simulink model "ModelSupervisor"  (R2017b)
settings: Solver=ode3  StartTime=0.0  StopTime=T_max  FixedStep=h  RelTol=1e-3
values from neighbouring files (symbols this model uses):
  b = 0.1    [Input_LQR.m]    (also in TestKalman.m; TestSuper.m; TestVahidComparison.m; parameter.m)
  C_sup = [1 0 0 0 0 0 ... (first row only)    [TestSuper.m]
  delta = cell(1,length(L_sup))    [TestSuper.m]
  g = 9.81    [Input_LQR.m]    (also in TestKalman.m; TestSuper.m; TestVahidComparison.m; parameter.m = 9.8)
  gamma = cell(1,length(L_sup))    [TestSuper.m]
  h = 0.01    [Input_LQR.m]    (also in TestKalman.m; TestSuper.m = 0.001; TestVahidComparison.m = 0.001; parameter.m)
  K = lqr(A, B, Q, R)    [Input_LQR.m]    (also in TestKalman.m; TestSuper.m)
  k = 0.15    [Input_LQR.m]    (also in TestKalman.m; TestSuper.m; TestVahidComparison.m; parameter.m)
  L = 1.4    [Input_LQR.m]    (also in TestKalman.m; TestSuper.m = 1.025; TestVahidComparison.m)
  L_2 = 1.525    [TestSuper.m]
  M = 1    [Input_LQR.m]    (also in TestKalman.m; TestSuper.m; TestVahidComparison.m; parameter.m)
  m = 3/4    (= 0.75)    [Input_LQR.m]    (also in TestKalman.m; TestSuper.m; TestVahidComparison.m; parameter.m)
  P_0 = diag([1,1,1,1,100,100])    [Input_LQR.m]    (also in TestKalman.m = diag([1,1,1,1,100,100])*0.001; TestSuper.m = diag([1,1,1,1,100,100])*0.001)
  phi = cell(1,length(L_sup))    [TestSuper.m]
  Q_kalman = diag([10, 10e-4])    [Input_LQR.m]    (also in TestKalman.m = diag([(10), (10e-4)]); TestSuper.m = diag([(10), (10e-4)]))
  R_kalman = diag([(10e-7), (10e-7)])    [Input_LQR.m]    (also in TestKalman.m; TestSuper.m)
  R_sup = R_kalman    [TestSuper.m]
  sys1 = c2d(ss(A_kA1, B_kA1, C_kA1, D_kA1), h)    [TestSuper.m]
  sys2 = c2d(ss(A_kA2, B_kA2, C_kA2, D_kA2), h)    [TestSuper.m]
  sys3 = c2d(ss(A_kA3, B_kA3, C_kA3, D_kA3), h)    [TestSuper.m]
  sys4 = c2d(ss(A_kA4, B_kA4, C_kA4, D_kA4), h)    [TestSuper.m]
  theta_0 = 0    [Input_LQR.m]    (also in TestKalman.m = 0.1; TestSuper.m = 0.1; TestVahidComparison.m = 0.1)
  theta_dot0 = 0    [Input_LQR.m]    (also in TestKalman.m; TestSuper.m; TestVahidComparison.m)
  X_0 = [0 0 0 0 0 0]'    [Input_LQR.m]    (also in TestKalman.m = [x_0 theta_0 x_dot0 theta_dot0 0 0]'; TestSuper.m = [x_0 theta_0 x_dot0 theta_dot0 0 0]')
  x_0 = 0    [Input_LQR.m]    (also in TestKalman.m; TestSuper.m; TestVahidComparison.m)
  x_dot0 = 0    [Input_LQR.m]    (also in TestKalman.m; TestSuper.m; TestVahidComparison.m)
  y_0 = [0 0]    [Input_LQR.m]    (also in TestKalman.m; TestSuper.m)
undefined symbols (not defined in the file or in its folder): A_kA1, A_kA2, A_kA3, A_kA4, B_kA1, B_kA2, B_kA3, B_kA4, C_kA1, C_kA2, C_kA3, C_kA4, D_kA1, D_kA2, D_kA3, D_kA4
libraries: simulink x6
settings Model: Creator=Erik  LastModifiedBy=Andreas
settings DataIOCC: LimitDataPoints=on  SaveFormat=Array
settings OptimizationCC: BlockReduction=off  BooleanDataType=off  LifeSpan=inf
settings DebuggingCC: SaveWithParameterizedLinksMsg=none  UnderspecifiedInitializationDetection=Classic  MergeDetectMultiDrivingBlocksExec=none  SignalResolutionControl=TryResolveAllWithWarning  SFUnexpectedBacktrackingDiag=warning  SFNoUnconditionalDefaultTransitionDiag=warning  SFExecutionAtInitializationDiag=none
settings HardwareCC: ProdBitPerPointer=32  ProdBitPerSizeT=32  ProdBitPerPtrDiffT=32  ProdLargestAtomicFloat=None  ProdIntDivRoundTo=Undefined  ProdEndianess=Unspecified  ProdWordSize=32  ProdHWDeviceType=32-bit Generic  TargetUnknown=on
settings ModelReferenceCC: PropagateSignalLabelsOutOfModel=off
settings CodeAppCC: StateflowObjectComments=on
settings GRTTargetCC: TargetLangStandard=C89/C90 (ANSI)  GeneratePreprocessorConditionals=Disable all
settings ConfigComp: CovMetricSettings=dw  CovHtmlReporting=on  CovSaveCumulativeToWorkspaceVar=on  CovSaveSingleToWorkspaceVar=on  CovExternalEMLEnable=off  CovSFcnEnable=off

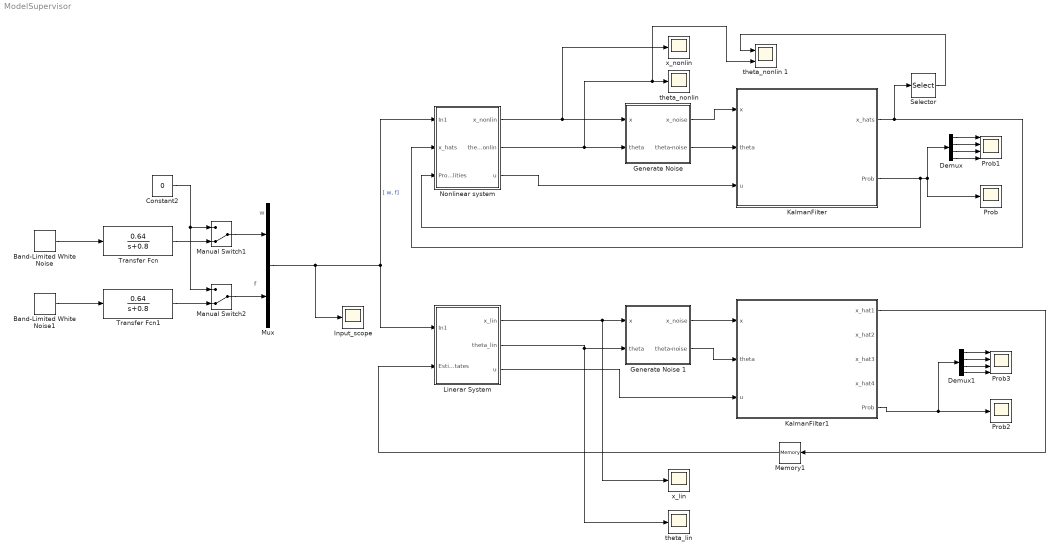
== system ModelSupervisor ==
  note: f
  note: w
  Band-Limited White Noise : simulink/Sources/Band-Limited White Noise  Cov=Q_kalman(1,1)  Ts=h  seed=[23343]
  Band-Limited White Noise1 : simulink/Sources/Band-Limited White Noise  Cov=Q_kalman(2,2)  Ts=h  seed=[23344]
  Constant2 : Constant  Value=0
  Demux : Demux
  Demux1 : Demux
  "Generate Noise " : Subsystem
  Generate Noise 1 : Subsystem
  Input_scope : Scope
  KalmanFilter : Subsystem
  KalmanFilter1 : Subsystem
  Linerar System : Subsystem
  Manual Switch1 : ManualSwitch  CurrentSetting=0
  Manual Switch2 : ManualSwitch  CurrentSetting=0
  Memory1 : Memory  InitialCondition=X_0
  Mux : Mux  Inputs=2
  "Nonlinear system " : Subsystem
  Prob : Scope
  Prob1 : Scope  NumInputPorts=4
  Prob2 : Scope
  Prob3 : Scope  NumInputPorts=4
  Selector : Selector  InputPortWidth=24  IndexOptions=Index vector (dialog)  Indices=[2 7 13 19]  OutputSizes=1
  Transfer Fcn : TransferFcn  Numerator=[0.64]  Denominator=[1 0.8]
  Transfer Fcn1 : TransferFcn  Numerator=[0.64]  Denominator=[1 0.8]
  theta_lin : Scope
  "theta_nonlin " : Scope
  theta_nonlin 1 : Scope  NumInputPorts=2
  x_lin : Scope
  x_nonlin : Scope
  wires:
  Mux/1 -> Linerar System/1(In1), "Nonlinear system "/1(In1), Input_scope/1  "[ w, f]"
  "Nonlinear system "/1(x_nonlin) -> x_nonlin/1, "Generate Noise "/1(x)
  "Nonlinear system "/2(theta_nonlin) -> theta_nonlin 1/2, "theta_nonlin "/1, "Generate Noise "/2(theta)
  Linerar System/2(theta_lin) -> theta_lin/1, Generate Noise 1/2(theta)
  "Nonlinear system "/3(u) -> KalmanFilter/3("u ")
  KalmanFilter/1(x_hats) -> Selector/1, "Nonlinear system "/2(x_hats)
  Band-Limited White Noise/1 -> Transfer Fcn/1
  Band-Limited White Noise1/1 -> Transfer Fcn1/1
  Transfer Fcn/1 -> Manual Switch1/2
  "Generate Noise "/1(x_noise) -> KalmanFilter/1(x)
  "Generate Noise "/2(theta-noise) -> KalmanFilter/2(theta)
  Generate Noise 1/2(theta-noise) -> KalmanFilter1/2(theta)
  Linerar System/3(u) -> KalmanFilter1/3("u ")
  Linerar System/1(x_lin) -> x_lin/1, Generate Noise 1/1(x)
  Generate Noise 1/1(x_noise) -> KalmanFilter1/1(x)
  Memory1/1 -> Linerar System/2(Estimated states)
  KalmanFilter/2(Prob) -> "Nonlinear system "/3(Probabilities), Prob/1, Demux/1
  KalmanFilter1/1(x_hat1) -> Memory1/1
  Demux/1 -> Prob1/1
  Demux/2 -> Prob1/2
  Demux/3 -> Prob1/3
  Demux/4 -> Prob1/4
  KalmanFilter1/5(Prob) -> Demux1/1, Prob2/1
  Demux1/1 -> Prob3/1
  Demux1/2 -> Prob3/2
  Demux1/3 -> Prob3/3
  Demux1/4 -> Prob3/4
  Manual Switch1/1 -> Mux/1
  Constant2/1 -> Manual Switch2/1, Manual Switch1/1
  Transfer Fcn1/1 -> Manual Switch2/2
  Manual Switch2/1 -> Mux/2
  Selector/1 -> theta_nonlin 1/1

== system ModelSupervisor/Generate Noise  ==
  x : Inport
  theta : Inport  Port=2
  Band-Limited White Noise2 : simulink/Sources/Band-Limited White Noise  Cov=R_kalman(1,1)  Ts=h  seed=[23342]
  Band-Limited White Noise3 : simulink/Sources/Band-Limited White Noise  Cov=R_kalman(2,2)  Ts=h  seed=[23341]
  Constant : Constant  Value=0
  Manual Switch : ManualSwitch  CurrentSetting=0
  Manual Switch1 : ManualSwitch  CurrentSetting=0
  Sum : Sum  Inputs=++|
  Sum1 : Sum  Inputs=|++
  x_noise : Outport
  theta-noise : Outport  Port=2
  wires:
  Sum/1 -> x_noise/1
  x/1 -> Sum/2
  Band-Limited White Noise2/1 -> Manual Switch1/1
  theta/1 -> Sum1/1
  Sum1/1 -> theta-noise/1
  Band-Limited White Noise3/1 -> Manual Switch/1
  Manual Switch/1 -> Sum1/2
  Manual Switch1/1 -> Sum/1
  Constant/1 -> Manual Switch/2, Manual Switch1/2

== system ModelSupervisor/Generate Noise 1 ==
  x : Inport
  theta : Inport  Port=2
  Band-Limited White Noise2 : simulink/Sources/Band-Limited White Noise  Cov=R_kalman(1,1)  Ts=h  seed=[23342]
  Band-Limited White Noise3 : simulink/Sources/Band-Limited White Noise  Cov=R_kalman(2,2)  Ts=h  seed=[23341]
  Sum : Sum  Inputs=++|
  Sum1 : Sum  Inputs=|++
  x_noise : Outport
  theta-noise : Outport  Port=2
  wires:
  Sum/1 -> x_noise/1
  x/1 -> Sum/2
  Band-Limited White Noise2/1 -> Sum/1
  theta/1 -> Sum1/1
  Sum1/1 -> theta-noise/1
  Band-Limited White Noise3/1 -> Sum1/2

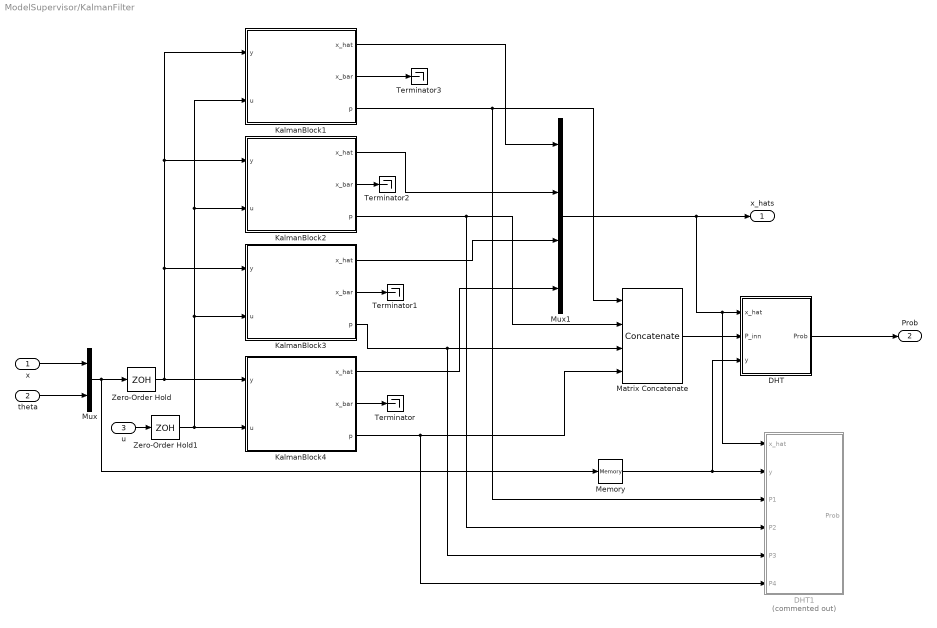
== system ModelSupervisor/KalmanFilter ==
  x : Inport
  theta : Inport  Port=2
  "u " : Inport  Port=3
  DHT : Subsystem
  DHT1 : Subsystem  Commented=on
  KalmanBlock1 : Subsystem
  KalmanBlock2 : Subsystem
  KalmanBlock3 : Subsystem
  KalmanBlock4 : Subsystem
  Matrix Concatenate : Concatenate  NumInputs=4  Mode=Multidimensional array  ConcatenateDimension=2
  Memory : Memory  InitialCondition=[x_0 theta_0]
  Mux : Mux  Inputs=2
  Mux1 : Mux
  Terminator{,1..3} (4 alike) : Terminator
  Zero-Order Hold : ZeroOrderHold  SampleTime=h
  Zero-Order Hold1 : ZeroOrderHold  SampleTime=h
  x_hats : Outport
  Prob : Outport  Port=2
  wires:
  Mux/1 -> Zero-Order Hold/1, Memory/1
  "u "/1 -> Zero-Order Hold1/1
  x/1 -> Mux/1
  theta/1 -> Mux/2
  KalmanBlock4/2(x_bar) -> Terminator/1
  KalmanBlock3/2(x_bar) -> Terminator1/1
  KalmanBlock2/2(x_bar) -> Terminator2/1
  KalmanBlock1/2(x_bar) -> Terminator3/1
  KalmanBlock1/1(x_hat) -> Mux1/1
  KalmanBlock2/1(x_hat) -> Mux1/2
  KalmanBlock3/1(x_hat) -> Mux1/3
  KalmanBlock4/1(x_hat) -> Mux1/4
  DHT/1(Prob) -> Prob/1
  Mux1/1 -> x_hats/1, DHT1/1(x_hat), DHT/1(x_hat)
  KalmanBlock3/3(p) -> DHT1/5(P3), Matrix Concatenate/3
  KalmanBlock2/3(p) -> DHT1/4(P2), Matrix Concatenate/2
  KalmanBlock1/3(p) -> DHT1/3(P1), Matrix Concatenate/1
  Matrix Concatenate/1 -> DHT/2(P_inn)
  Memory/1 -> DHT1/2(y), DHT/3(y)
  KalmanBlock4/3(p) -> DHT1/6(P4), Matrix Concatenate/4
  Zero-Order Hold/1 -> KalmanBlock1/1("y "), KalmanBlock2/1("y "), KalmanBlock3/1("y "), KalmanBlock4/1("y ")
  Zero-Order Hold1/1 -> KalmanBlock1/2("u "), KalmanBlock2/2("u "), KalmanBlock3/2("u "), KalmanBlock4/2("u ")

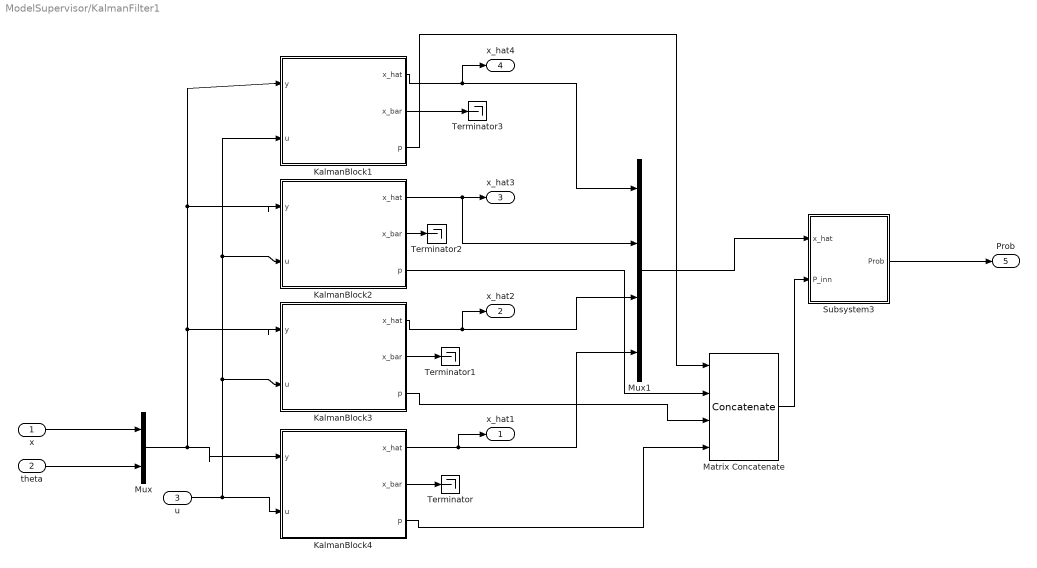
== system ModelSupervisor/KalmanFilter1 ==
  x : Inport
  theta : Inport  Port=2
  "u " : Inport  Port=3
  KalmanBlock1 : Subsystem
  KalmanBlock2 : Subsystem
  KalmanBlock3 : Subsystem
  KalmanBlock4 : Subsystem
  Matrix Concatenate : Concatenate  NumInputs=4  Mode=Multidimensional array  ConcatenateDimension=2
  Mux : Mux  Inputs=2
  Mux1 : Mux
  Subsystem3 : Subsystem
  Terminator{,1..3} (4 alike) : Terminator
  x_hat1 : Outport
  x_hat2 : Outport  Port=2
  x_hat3 : Outport  Port=3
  x_hat4 : Outport  Port=4
  Prob : Outport  Port=5
  wires:
  Mux/1 -> KalmanBlock1/1("y "), KalmanBlock2/1("y "), KalmanBlock3/1("y "), KalmanBlock4/1("y ")
  "u "/1 -> KalmanBlock3/2("u "), KalmanBlock2/2("u "), KalmanBlock1/2("u "), KalmanBlock4/2("u ")
  x/1 -> Mux/1
  theta/1 -> Mux/2
  KalmanBlock4/2(x_bar) -> Terminator/1
  KalmanBlock3/2(x_bar) -> Terminator1/1
  KalmanBlock2/2(x_bar) -> Terminator2/1
  KalmanBlock1/2(x_bar) -> Terminator3/1
  KalmanBlock1/1(x_hat) -> Mux1/1, x_hat4/1
  KalmanBlock2/1(x_hat) -> x_hat3/1, Mux1/2
  KalmanBlock3/1(x_hat) -> Mux1/3, x_hat2/1
  KalmanBlock4/1(x_hat) -> Mux1/4, x_hat1/1
  Subsystem3/1(Prob) -> Prob/1
  Mux1/1 -> Subsystem3/1(x_hat)
  KalmanBlock4/3(p) -> Matrix Concatenate/4
  KalmanBlock3/3(p) -> Matrix Concatenate/3
  KalmanBlock2/3(p) -> Matrix Concatenate/2
  KalmanBlock1/3(p) -> Matrix Concatenate/1
  Matrix Concatenate/1 -> Subsystem3/2(P_inn)

== system ModelSupervisor/Linerar System ==
  In1 : Inport
  Estimated states : Inport  Port=2
  Demux : Demux  Outputs=2
  LQR : Subsystem
  "theta system " : Subsystem
  x system : Subsystem
  x_lin : Outport
  theta_lin : Outport  Port=2
  u : Outport  Port=3
  wires:
  x system/1(x) -> "theta system "/4(x), x_lin/1
  Demux/1 -> "theta system "/2(w), x system/2(w)
  "theta system "/1(theta) -> theta_lin/1, x system/3(theta)
  Demux/2 -> "theta system "/3(f)
  x system/2(x_dot) -> "theta system "/5(x_dot)
  In1/1 -> Demux/1
  LQR/1(u) -> u/1, "theta system "/1("u "), x system/1("u ")
  Estimated states/1 -> LQR/1(x)

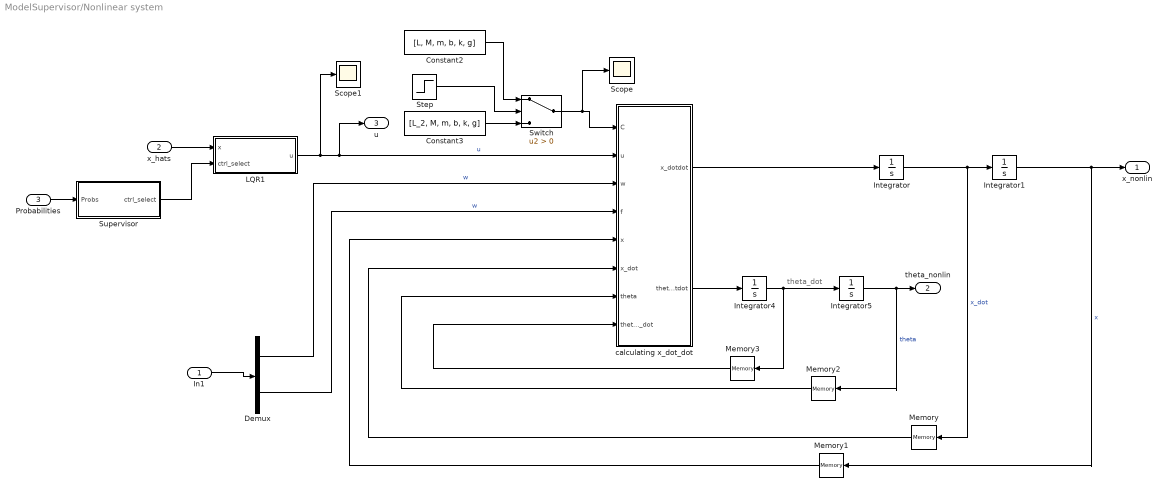
== system ModelSupervisor/Nonlinear system  ==
  note: theta_dot
  In1 : Inport
  x_hats : Inport  Port=2
  Probabilities : Inport  Port=3
  Constant2 : Constant  Value=[L, M, m, b, k, g]  SampleTime=0.01
  Constant3 : Constant  Value=[L_2, M, m, b, k, g]  SampleTime=0.01
  Demux : Demux  Outputs=2
  Integrator : Integrator  InitialCondition=x_dot0
  Integrator1 : Integrator  InitialCondition=x_0
  Integrator4 : Integrator  InitialCondition=theta_dot0
  Integrator5 : Integrator  InitialCondition=theta_0
  LQR1 : Subsystem
  Memory : Memory  InitialCondition=x_dot0
  Memory1 : Memory  InitialCondition=x_0
  Memory2 : Memory  InitialCondition=theta_0
  Memory3 : Memory  InitialCondition=theta_dot0
  Scope : Scope
  Scope1 : Scope
  Step : Step  Time=10  Before=-1  SampleTime=0
  Supervisor : Subsystem
  Switch : Switch  Criteria=u2 > Threshold
  calculating x_dot_dot : MATLAB Function  TreatAsAtomicUnit=on
  x_nonlin : Outport
  theta_nonlin : Outport  Port=2
  u : Outport  Port=3
  wires:
  In1/1 -> Demux/1
  LQR1/1(u) -> Scope1/1, u/1, calculating x_dot_dot/2(u)  "u"
  Demux/1 -> calculating x_dot_dot/3(w)  "w"
  calculating x_dot_dot/1(x_dotdot) -> Integrator/1
  Integrator/1 -> Memory/1, Integrator1/1  "x_dot"
  Integrator1/1 -> Memory1/1, x_nonlin/1  "x"
  calculating x_dot_dot/2(theta_dotdot) -> Integrator4/1
  Integrator4/1 -> Memory3/1, Integrator5/1
  Integrator5/1 -> Memory2/1, theta_nonlin/1  "theta"
  Memory1/1 -> calculating x_dot_dot/5(x)
  Memory/1 -> calculating x_dot_dot/6(x_dot)
  Memory2/1 -> calculating x_dot_dot/7(theta)
  Memory3/1 -> calculating x_dot_dot/8(theta_dot)
  Demux/2 -> calculating x_dot_dot/4(f)  "w"
  Supervisor/1(ctrl_select) -> LQR1/2(ctrl_select)
  Probabilities/1 -> Supervisor/1(Probs)
  x_hats/1 -> LQR1/1(x)
  Constant2/1 -> Switch/1
  Step/1 -> Switch/2
  Constant3/1 -> Switch/3
  Switch/1 -> Scope/1, calculating x_dot_dot/1(C)

== system ModelSupervisor/KalmanFilter/DHT ==
  x_hat : Inport
  P_inn : Inport  Port=2
  y : Inport  Port=3
  Constant : Constant  Value=C_sup
  Constant1 : Constant  Value=R_sup
  MATLAB Function : MATLAB Function  TreatAsAtomicUnit=on
  Memory : Memory  InitialCondition=[1/4 1/4 1/4 1/4]'
  Prob : Outport  PortDimensions=[4]
  wires:
  MATLAB Function/1(Prob) -> Memory/1
  P_inn/1 -> MATLAB Function/5(P)
  x_hat/1 -> MATLAB Function/1(x_hat)
  Constant/1 -> MATLAB Function/3(C)
  Constant1/1 -> MATLAB Function/4(R)
  Memory/1 -> Prob/1, MATLAB Function/6(Prob_prev)
  y/1 -> MATLAB Function/2(y)

== system ModelSupervisor/KalmanFilter/DHT1 ==
  x_hat : Inport
  y : Inport  Port=2
  P1 : Inport  Port=3
  P2 : Inport  Port=4
  P3 : Inport  Port=5
  P4 : Inport  Port=6
  Constant : Constant  Value=C_sup
  Constant1 : Constant  Value=R_sup
  Demux : Demux
  MATLAB Function : MATLAB Function  TreatAsAtomicUnit=on
  Memory : Memory  InitialCondition=[1/4 1/4 1/4 1/4]'
  Scope : Scope  NumInputPorts=4
  Scope1 : Scope
  Prob : Outport  PortDimensions=[4]
  wires:
  MATLAB Function/1(Prob) -> Memory/1
  x_hat/1 -> MATLAB Function/1(x_hat)
  Constant/1 -> MATLAB Function/3(C)
  Constant1/1 -> MATLAB Function/4(R)
  Memory/1 -> MATLAB Function/9(Prob_prev), Prob/1
  y/1 -> MATLAB Function/2("y ")
  P2/1 -> MATLAB Function/6(P2)
  P1/1 -> MATLAB Function/5(P1)
  P3/1 -> MATLAB Function/7(P3)
  P4/1 -> MATLAB Function/8(P4)
  Demux/1 -> Scope/1
  Demux/2 -> Scope/2
  Demux/4 -> Scope/4
  Demux/3 -> Scope/3
  MATLAB Function/2(Prob_0) -> Demux/1
  MATLAB Function/3(y) -> Scope1/1

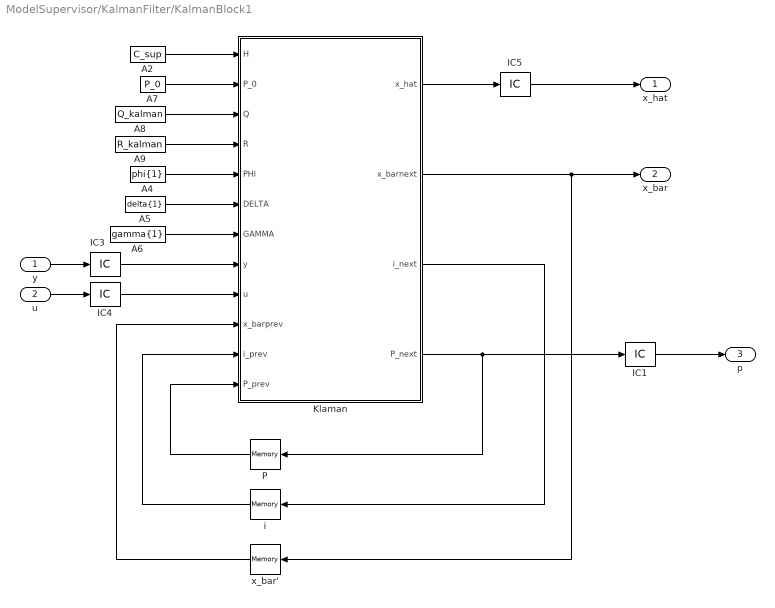
== system ModelSupervisor/KalmanFilter/KalmanBlock1 ==
  "y " : Inport
  "u " : Inport  Port=2
  A2 : Constant  Value=C_sup
  A4 : Constant  Value=phi{1}
  A5 : Constant  Value=delta{1}
  A6 : Constant  Value=gamma{1}
  A7 : Constant  Value=P_0
  A8 : Constant  Value=Q_kalman
  A9 : Constant  Value=R_kalman
  IC1 : InitialCondition  Value=P_0
  IC3 : InitialCondition  Value=y_0
  IC4 : InitialCondition  Value=0
  IC5 : InitialCondition  Value=X_0
  Klaman : MATLAB Function  TreatAsAtomicUnit=on
  P : Memory  InitialCondition=P_0
  "i " : Memory
  x_bar' : Memory  InitialCondition=X_0
  x_hat : Outport
  x_bar : Outport  Port=2
  p : Outport  Port=3
  wires:
  A8/1 -> Klaman/3(Q)
  A6/1 -> Klaman/7(GAMMA)
  A4/1 -> Klaman/5(PHI)
  Klaman/2(x_barnext) -> x_bar'/1, x_bar/1
  Klaman/3(i_next) -> "i "/1
  Klaman/1(x_hat) -> IC5/1
  A2/1 -> Klaman/1(H)
  A5/1 -> Klaman/6(DELTA)
  IC4/1 -> Klaman/9(u)
  A7/1 -> Klaman/2(P_0)
  "u "/1 -> IC4/1
  A9/1 -> Klaman/4(R)
  "y "/1 -> IC3/1
  IC5/1 -> x_hat/1
  IC3/1 -> Klaman/8(y)
  "i "/1 -> Klaman/11(i_prev)
  P/1 -> Klaman/12(P_prev)
  x_bar'/1 -> Klaman/10(x_barprev)
  Klaman/4(P_next) -> P/1, IC1/1
  IC1/1 -> p/1

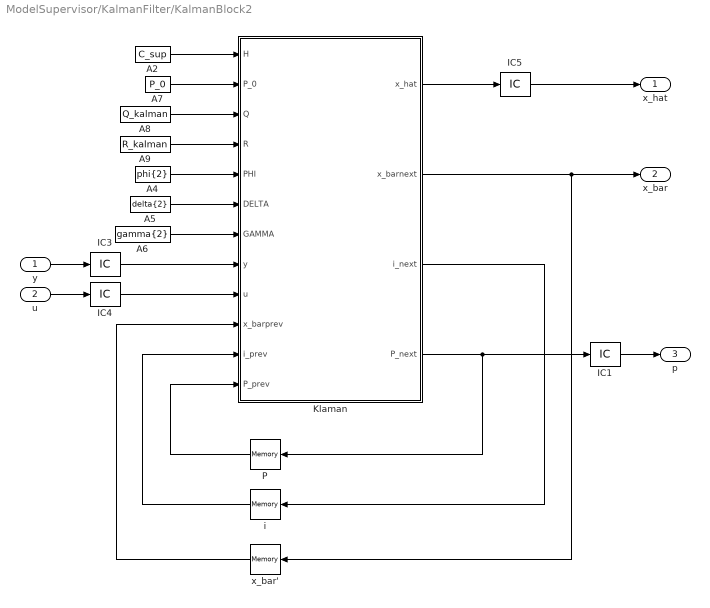
== system ModelSupervisor/KalmanFilter/KalmanBlock2 ==
  "y " : Inport
  "u " : Inport  Port=2
  A2 : Constant  Value=C_sup
  A4 : Constant  Value=phi{2}
  A5 : Constant  Value=delta{2}
  A6 : Constant  Value=gamma{2}
  A7 : Constant  Value=P_0
  A8 : Constant  Value=Q_kalman
  A9 : Constant  Value=R_kalman
  IC1 : InitialCondition  Value=P_0
  IC3 : InitialCondition  Value=y_0
  IC4 : InitialCondition  Value=0
  IC5 : InitialCondition  Value=X_0
  Klaman : MATLAB Function  TreatAsAtomicUnit=on
  P : Memory  InitialCondition=P_0
  "i " : Memory
  x_bar' : Memory  InitialCondition=X_0
  x_hat : Outport
  x_bar : Outport  Port=2
  p : Outport  Port=3
  wires:
  Klaman/2(x_barnext) -> x_bar'/1, x_bar/1
  Klaman/3(i_next) -> "i "/1
  Klaman/1(x_hat) -> IC5/1
  IC4/1 -> Klaman/9(u)
  "u "/1 -> IC4/1
  "y "/1 -> IC3/1
  IC5/1 -> x_hat/1
  IC3/1 -> Klaman/8(y)
  "i "/1 -> Klaman/11(i_prev)
  P/1 -> Klaman/12(P_prev)
  x_bar'/1 -> Klaman/10(x_barprev)
  Klaman/4(P_next) -> IC1/1, P/1
  A8/1 -> Klaman/3(Q)
  A6/1 -> Klaman/7(GAMMA)
  A4/1 -> Klaman/5(PHI)
  A2/1 -> Klaman/1(H)
  A5/1 -> Klaman/6(DELTA)
  A7/1 -> Klaman/2(P_0)
  A9/1 -> Klaman/4(R)
  IC1/1 -> p/1

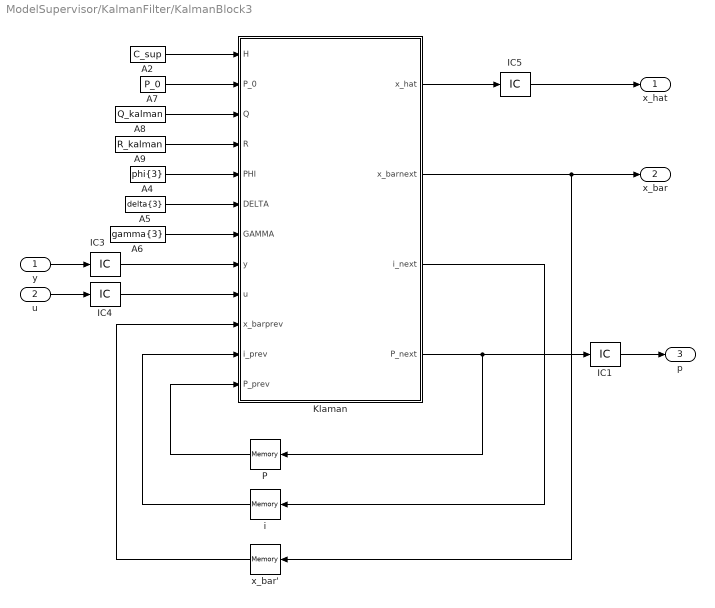
== system ModelSupervisor/KalmanFilter/KalmanBlock3 ==
  "y " : Inport
  "u " : Inport  Port=2
  A2 : Constant  Value=C_sup
  A4 : Constant  Value=phi{3}
  A5 : Constant  Value=delta{3}
  A6 : Constant  Value=gamma{3}
  A7 : Constant  Value=P_0
  A8 : Constant  Value=Q_kalman
  A9 : Constant  Value=R_kalman
  IC1 : InitialCondition  Value=P_0
  IC3 : InitialCondition  Value=y_0
  IC4 : InitialCondition  Value=0
  IC5 : InitialCondition  Value=X_0
  Klaman : MATLAB Function  TreatAsAtomicUnit=on
  P : Memory  InitialCondition=P_0
  "i " : Memory
  x_bar' : Memory  InitialCondition=X_0
  x_hat : Outport
  x_bar : Outport  Port=2
  p : Outport  Port=3
  wires:
  Klaman/2(x_barnext) -> x_bar'/1, x_bar/1
  Klaman/3(i_next) -> "i "/1
  Klaman/1(x_hat) -> IC5/1
  IC4/1 -> Klaman/9(u)
  "u "/1 -> IC4/1
  "y "/1 -> IC3/1
  IC5/1 -> x_hat/1
  IC3/1 -> Klaman/8(y)
  "i "/1 -> Klaman/11(i_prev)
  P/1 -> Klaman/12(P_prev)
  x_bar'/1 -> Klaman/10(x_barprev)
  Klaman/4(P_next) -> IC1/1, P/1
  A8/1 -> Klaman/3(Q)
  A6/1 -> Klaman/7(GAMMA)
  A4/1 -> Klaman/5(PHI)
  A2/1 -> Klaman/1(H)
  A5/1 -> Klaman/6(DELTA)
  A7/1 -> Klaman/2(P_0)
  A9/1 -> Klaman/4(R)
  IC1/1 -> p/1

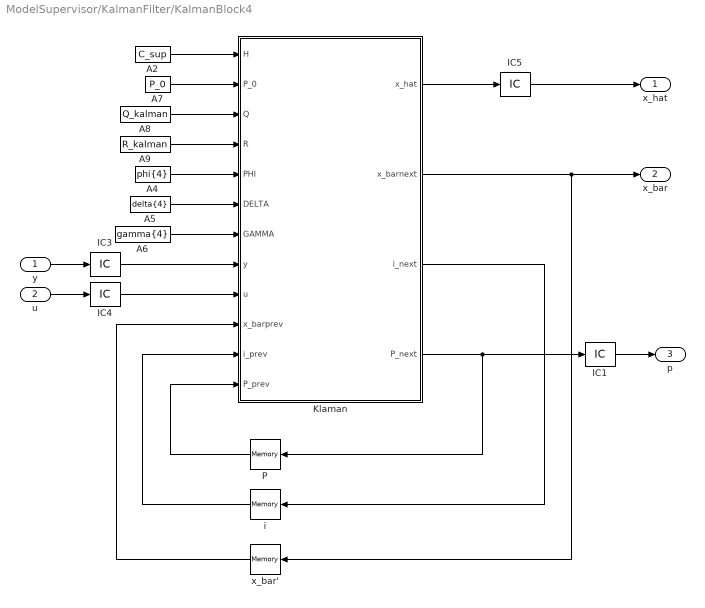
== system ModelSupervisor/KalmanFilter/KalmanBlock4 ==
  "y " : Inport
  "u " : Inport  Port=2
  A2 : Constant  Value=C_sup
  A4 : Constant  Value=phi{4}
  A5 : Constant  Value=delta{4}
  A6 : Constant  Value=gamma{4}
  A7 : Constant  Value=P_0
  A8 : Constant  Value=Q_kalman
  A9 : Constant  Value=R_kalman
  IC1 : InitialCondition  Value=P_0
  IC3 : InitialCondition  Value=y_0
  IC4 : InitialCondition  Value=0
  IC5 : InitialCondition  Value=X_0
  Klaman : MATLAB Function  TreatAsAtomicUnit=on
  P : Memory  InitialCondition=P_0
  "i " : Memory
  x_bar' : Memory  InitialCondition=X_0
  x_hat : Outport
  x_bar : Outport  Port=2
  p : Outport  Port=3
  wires:
  Klaman/2(x_barnext) -> x_bar'/1, x_bar/1
  Klaman/3(i_next) -> "i "/1
  Klaman/1(x_hat) -> IC5/1
  Klaman/4(P_next) -> P/1, IC1/1
  IC4/1 -> Klaman/9(u)
  "u "/1 -> IC4/1
  "y "/1 -> IC3/1
  IC5/1 -> x_hat/1
  IC3/1 -> Klaman/8(y)
  "i "/1 -> Klaman/11(i_prev)
  P/1 -> Klaman/12(P_prev)
  x_bar'/1 -> Klaman/10(x_barprev)
  A8/1 -> Klaman/3(Q)
  A6/1 -> Klaman/7(GAMMA)
  A4/1 -> Klaman/5(PHI)
  A2/1 -> Klaman/1(H)
  A5/1 -> Klaman/6(DELTA)
  A7/1 -> Klaman/2(P_0)
  A9/1 -> Klaman/4(R)
  IC1/1 -> p/1

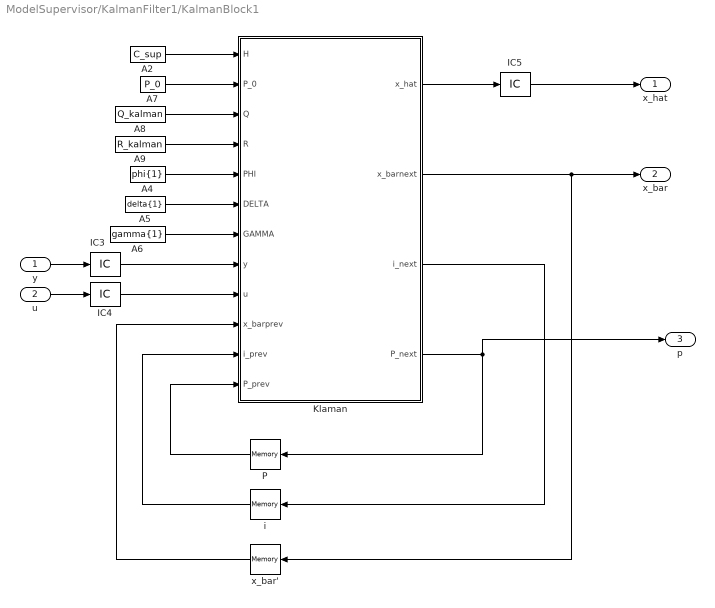
== system ModelSupervisor/KalmanFilter1/KalmanBlock1 ==
  "y " : Inport
  "u " : Inport  Port=2
  A2 : Constant  Value=C_sup
  A4 : Constant  Value=phi{1}
  A5 : Constant  Value=delta{1}
  A6 : Constant  Value=gamma{1}
  A7 : Constant  Value=P_0
  A8 : Constant  Value=Q_kalman
  A9 : Constant  Value=R_kalman
  IC3 : InitialCondition  Value=y_0
  IC4 : InitialCondition  Value=0
  IC5 : InitialCondition  Value=X_0
  Klaman : MATLAB Function  TreatAsAtomicUnit=on
  P : Memory  InitialCondition=P_0
  "i " : Memory
  x_bar' : Memory  InitialCondition=X_0
  x_hat : Outport
  x_bar : Outport  Port=2
  p : Outport  Port=3
  wires:
  A8/1 -> Klaman/3(Q)
  A6/1 -> Klaman/7(GAMMA)
  A4/1 -> Klaman/5(PHI)
  Klaman/2(x_barnext) -> x_bar'/1, x_bar/1
  Klaman/3(i_next) -> "i "/1
  Klaman/1(x_hat) -> IC5/1
  A2/1 -> Klaman/1(H)
  A5/1 -> Klaman/6(DELTA)
  IC4/1 -> Klaman/9(u)
  A7/1 -> Klaman/2(P_0)
  "u "/1 -> IC4/1
  A9/1 -> Klaman/4(R)
  "y "/1 -> IC3/1
  IC5/1 -> x_hat/1
  IC3/1 -> Klaman/8(y)
  "i "/1 -> Klaman/11(i_prev)
  P/1 -> Klaman/12(P_prev)
  x_bar'/1 -> Klaman/10(x_barprev)
  Klaman/4(P_next) -> P/1, p/1

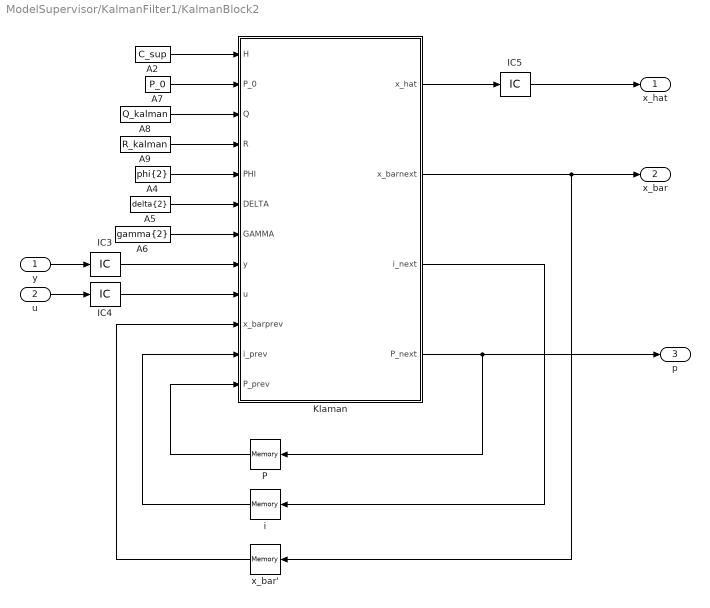
== system ModelSupervisor/KalmanFilter1/KalmanBlock2 ==
  "y " : Inport
  "u " : Inport  Port=2
  A2 : Constant  Value=C_sup
  A4 : Constant  Value=phi{2}
  A5 : Constant  Value=delta{2}
  A6 : Constant  Value=gamma{2}
  A7 : Constant  Value=P_0
  A8 : Constant  Value=Q_kalman
  A9 : Constant  Value=R_kalman
  IC3 : InitialCondition  Value=y_0
  IC4 : InitialCondition  Value=0
  IC5 : InitialCondition  Value=X_0
  Klaman : MATLAB Function  TreatAsAtomicUnit=on
  P : Memory  InitialCondition=P_0
  "i " : Memory
  x_bar' : Memory  InitialCondition=X_0
  x_hat : Outport
  x_bar : Outport  Port=2
  p : Outport  Port=3
  wires:
  Klaman/2(x_barnext) -> x_bar'/1, x_bar/1
  Klaman/3(i_next) -> "i "/1
  Klaman/1(x_hat) -> IC5/1
  IC4/1 -> Klaman/9(u)
  "u "/1 -> IC4/1
  "y "/1 -> IC3/1
  IC5/1 -> x_hat/1
  IC3/1 -> Klaman/8(y)
  "i "/1 -> Klaman/11(i_prev)
  P/1 -> Klaman/12(P_prev)
  x_bar'/1 -> Klaman/10(x_barprev)
  Klaman/4(P_next) -> p/1, P/1
  A8/1 -> Klaman/3(Q)
  A6/1 -> Klaman/7(GAMMA)
  A4/1 -> Klaman/5(PHI)
  A2/1 -> Klaman/1(H)
  A5/1 -> Klaman/6(DELTA)
  A7/1 -> Klaman/2(P_0)
  A9/1 -> Klaman/4(R)

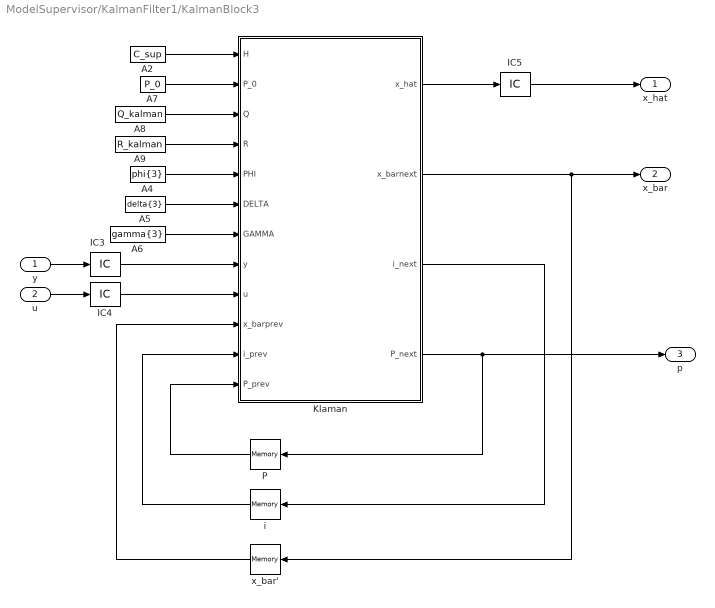
== system ModelSupervisor/KalmanFilter1/KalmanBlock3 ==
  "y " : Inport
  "u " : Inport  Port=2
  A2 : Constant  Value=C_sup
  A4 : Constant  Value=phi{3}
  A5 : Constant  Value=delta{3}
  A6 : Constant  Value=gamma{3}
  A7 : Constant  Value=P_0
  A8 : Constant  Value=Q_kalman
  A9 : Constant  Value=R_kalman
  IC3 : InitialCondition  Value=y_0
  IC4 : InitialCondition  Value=0
  IC5 : InitialCondition  Value=X_0
  Klaman : MATLAB Function  TreatAsAtomicUnit=on
  P : Memory  InitialCondition=P_0
  "i " : Memory
  x_bar' : Memory  InitialCondition=X_0
  x_hat : Outport
  x_bar : Outport  Port=2
  p : Outport  Port=3
  wires:
  Klaman/2(x_barnext) -> x_bar'/1, x_bar/1
  Klaman/3(i_next) -> "i "/1
  Klaman/1(x_hat) -> IC5/1
  IC4/1 -> Klaman/9(u)
  "u "/1 -> IC4/1
  "y "/1 -> IC3/1
  IC5/1 -> x_hat/1
  IC3/1 -> Klaman/8(y)
  "i "/1 -> Klaman/11(i_prev)
  P/1 -> Klaman/12(P_prev)
  x_bar'/1 -> Klaman/10(x_barprev)
  Klaman/4(P_next) -> p/1, P/1
  A8/1 -> Klaman/3(Q)
  A6/1 -> Klaman/7(GAMMA)
  A4/1 -> Klaman/5(PHI)
  A2/1 -> Klaman/1(H)
  A5/1 -> Klaman/6(DELTA)
  A7/1 -> Klaman/2(P_0)
  A9/1 -> Klaman/4(R)

== system ModelSupervisor/KalmanFilter1/KalmanBlock4 ==
  "y " : Inport
  "u " : Inport  Port=2
  A2 : Constant  Value=C_sup
  A4 : Constant  Value=phi{4}
  A5 : Constant  Value=delta{4}
  A6 : Constant  Value=gamma{4}
  A7 : Constant  Value=P_0
  A8 : Constant  Value=Q_kalman
  A9 : Constant  Value=R_kalman
  IC3 : InitialCondition  Value=y_0
  IC4 : InitialCondition  Value=0
  IC5 : InitialCondition  Value=X_0
  Klaman : MATLAB Function  TreatAsAtomicUnit=on
  P : Memory  InitialCondition=P_0
  "i " : Memory
  x_bar' : Memory  InitialCondition=X_0
  x_hat : Outport
  x_bar : Outport  Port=2
  p : Outport  Port=3
  wires:
  Klaman/2(x_barnext) -> x_bar'/1, x_bar/1
  Klaman/3(i_next) -> "i "/1
  Klaman/1(x_hat) -> IC5/1
  Klaman/4(P_next) -> P/1, p/1
  IC4/1 -> Klaman/9(u)
  "u "/1 -> IC4/1
  "y "/1 -> IC3/1
  IC5/1 -> x_hat/1
  IC3/1 -> Klaman/8(y)
  "i "/1 -> Klaman/11(i_prev)
  P/1 -> Klaman/12(P_prev)
  x_bar'/1 -> Klaman/10(x_barprev)
  A8/1 -> Klaman/3(Q)
  A6/1 -> Klaman/7(GAMMA)
  A4/1 -> Klaman/5(PHI)
  A2/1 -> Klaman/1(H)
  A5/1 -> Klaman/6(DELTA)
  A7/1 -> Klaman/2(P_0)
  A9/1 -> Klaman/4(R)

== system ModelSupervisor/KalmanFilter1/Subsystem3 ==
  x_hat : Inport
  P_inn : Inport  Port=2
  Constant : Constant  Value=C_sup
  Constant1 : Constant  Value=R_sup
  MATLAB Function : MATLAB Function  TreatAsAtomicUnit=on
  Memory : Memory  InitialCondition=[1/4 1/4 1/4 1/4]'
  Prob : Outport
  wires:
  MATLAB Function/1(Prob) -> Memory/1
  P_inn/1 -> MATLAB Function/4(P)
  x_hat/1 -> MATLAB Function/1(x_hat)
  Constant/1 -> MATLAB Function/2(C)
  Constant1/1 -> MATLAB Function/3(R)
  Memory/1 -> MATLAB Function/5(Prob_prev), Prob/1

== system ModelSupervisor/Linerar System/LQR ==
  x : Inport
  Gain : Gain  Gain=-K  Multiplication=Matrix(K*u)
  u : Outport
  wires:
  Gain/1 -> u/1
  x/1 -> Gain/1

== system ModelSupervisor/Linerar System/theta system  ==
  note: theta
  note: theta_dotdot
  note: theta_dot
  "u " : Inport
  w : Inport  Port=2
  f : Inport  Port=3
  x : Inport  Port=4
  x_dot : Inport  Port=5
  Constant : Constant  Value=[L M m b k g]  VectorParams1D=off  SampleTime=0.01
  Integrator : Integrator  InitialCondition=theta_dot0
  Integrator1 : Integrator  InitialCondition=theta_0
  MATLAB Function : MATLAB Function  TreatAsAtomicUnit=on
  Memory2 : Memory  InitialCondition=theta_0
  theta : Outport
  wires:
  MATLAB Function/1(theta_dotdot) -> Integrator/1
  "u "/1 -> MATLAB Function/1(u)
  w/1 -> MATLAB Function/2(w)
  x/1 -> MATLAB Function/4(x)
  Integrator1/1 -> Memory2/1, theta/1
  Constant/1 -> MATLAB Function/6(data)
  f/1 -> MATLAB Function/3(f)
  x_dot/1 -> MATLAB Function/5(x_dot)
  Memory2/1 -> MATLAB Function/7(theta)
  Integrator/1 -> Integrator1/1

== system ModelSupervisor/Linerar System/x system ==
  note: x
  note: x_dotdot
  note: x_dot
  "u " : Inport
  w : Inport  Port=2
  theta : Inport  Port=3
  Constant : Constant  Value=[L M m b k g]  VectorParams1D=off  SampleTime=0.01
  Integrator : Integrator  InitialCondition=x_dot0
  Integrator1 : Integrator  InitialCondition=x_0
  MATLAB Function : MATLAB Function  TreatAsAtomicUnit=on
  Memory1 : Memory  InitialCondition=x_dot0
  Memory2 : Memory  InitialCondition=x_0
  x : Outport
  x_dot : Outport  Port=2
  wires:
  Memory1/1 -> MATLAB Function/6(x_dot)
  "u "/1 -> MATLAB Function/1(u)
  w/1 -> MATLAB Function/2(w)
  theta/1 -> MATLAB Function/3(theta)
  Integrator1/1 -> Memory2/1, x/1
  Memory2/1 -> MATLAB Function/5(x)
  Constant/1 -> MATLAB Function/4(data)
  Integrator/1 -> Integrator1/1, x_dot/1, Memory1/1
  MATLAB Function/1(x_dotdot) -> Integrator/1

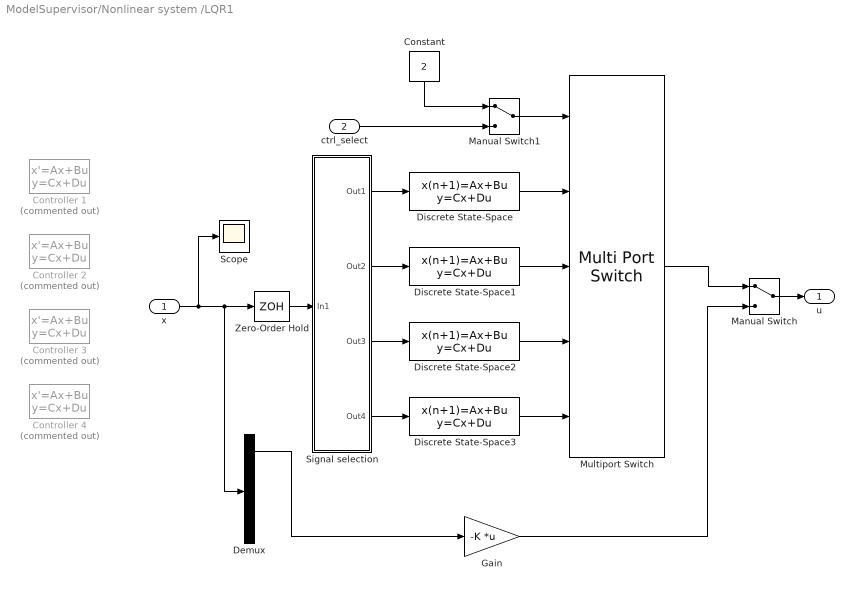
== system ModelSupervisor/Nonlinear system /LQR1 ==
  x : Inport
  ctrl_select : Inport  Port=2
  Constant : Constant  Value=2
  Controller 1 : StateSpace  Commented=on  A=A_kA1  B=B_kA1  C=C_kA1  D=D_kA1  InitialCondition=0
  Controller 2 : StateSpace  Commented=on  A=A_kA2  B=B_kA2  C=C_kA2  D=D_kA2  InitialCondition=0
  Controller 3 : StateSpace  Commented=on  A=A_kA3  B=B_kA3  C=C_kA3  D=D_kA3  InitialCondition=0
  Controller 4 : StateSpace  Commented=on  A=A_kA4  B=B_kA4  C=C_kA4  D=D_kA4  InitialCondition=0
  Demux : Demux
  Discrete State-Space : DiscreteStateSpace  A=sys1.A  B=sys1.B  C=sys1.C  D=sys1.D  SampleTime=h
  Discrete State-Space1 : DiscreteStateSpace  A=sys2.A  B=sys2.B  C=sys2.C  D=sys2.D  SampleTime=h
  Discrete State-Space2 : DiscreteStateSpace  A=sys3.A  B=sys3.B  C=sys3.C  D=sys3.D  SampleTime=h
  Discrete State-Space3 : DiscreteStateSpace  A=sys4.A  B=sys4.B  C=sys4.C  D=sys4.D  SampleTime=h
  Gain : Gain  Gain=-K  Multiplication=Matrix(K*u)
  Manual Switch : ManualSwitch
  Manual Switch1 : ManualSwitch
  Multiport Switch : MultiPortSwitch  Inputs=4
  Scope : Scope
  Signal selection : Subsystem
  Zero-Order Hold : ZeroOrderHold  SampleTime=h
  u : Outport
  wires:
  Demux/1 -> Gain/1
  Gain/1 -> Manual Switch/2
  Signal selection/1(Out1) -> Discrete State-Space/1
  Discrete State-Space/1 -> Multiport Switch/2
  Discrete State-Space1/1 -> Multiport Switch/3
  Signal selection/2(Out2) -> Discrete State-Space1/1
  Discrete State-Space2/1 -> Multiport Switch/4
  Signal selection/3(Out3) -> Discrete State-Space2/1
  Discrete State-Space3/1 -> Multiport Switch/5
  Signal selection/4(Out4) -> Discrete State-Space3/1
  Zero-Order Hold/1 -> Signal selection/1(In1)
  x/1 -> Scope/1, Demux/1, Zero-Order Hold/1
  Manual Switch/1 -> u/1
  Multiport Switch/1 -> Manual Switch/1
  Manual Switch1/1 -> Multiport Switch/1
  Constant/1 -> Manual Switch1/1
  ctrl_select/1 -> Manual Switch1/2

== system ModelSupervisor/Nonlinear system /Supervisor ==
  Probs : Inport
  Clock : Clock
  Memory : Memory  InitialCondition=-1
  Memory1 : Memory  InitialCondition=1
  Scope : Scope
  Supervisor : MATLAB Function  TreatAsAtomicUnit=on
  ctrl_select : Outport
  wires:
  Probs/1 -> Supervisor/1(probs)
  Supervisor/1(ctrl_selection) -> Scope/1, Memory1/1, ctrl_select/1
  Clock/1 -> Supervisor/2(current_time)
  Supervisor/2(last_change_time) -> Memory/1
  Memory/1 -> Supervisor/4("last_change_time ")
  Memory1/1 -> Supervisor/3(current_controller)

== system ModelSupervisor/Nonlinear system /LQR1/Signal selection ==
  In1 : Inport
  Demux : Demux
  Selector{,1..3} (4 alike) : Selector  InputPortWidth=6  IndexOptions=Index vector (dialog)  Indices=[2 1]  OutputSizes=1
  Out1 : Outport
  Out2 : Outport  Port=2
  Out3 : Outport  Port=3
  Out4 : Outport  Port=4
  wires:
  Selector/1 -> Out1/1
  Demux/2 -> Selector1/1
  In1/1 -> Demux/1
  Demux/3 -> Selector2/1
  Demux/1 -> Selector/1
  Demux/4 -> Selector3/1
  Selector3/1 -> Out4/1
  Selector2/1 -> Out3/1
  Selector1/1 -> Out2/1

== matlab function ModelSupervisor/Linerar System/x system/MATLAB Function ==
  data: u input; w input; theta input; data input; x_dotdot output; x input; x_dot input
function x_dotdot  = fcn(u, w, theta, data, x, x_dot)
L = data(1);
M = data(2);
m = data(3);
b = data(4);
k = data(5);
g = data(6);

% theta = theta * 180 / pi;

x_dotdot=(u - w - m * g * theta - b * x_dot - k * x) / M;


end

== matlab function ModelSupervisor/KalmanFilter/KalmanBlock4/Klaman ==
  data: H input; P_0 input; Q input; R input; PHI input; DELTA input; GAMMA input; y input; u input; x_barprev input; i_prev input; P_prev input; x_hat output; x_barnext output; i_next output; P_next output
function [x_hat,x_barnext,i_next,P_next] = KalmanFilter(H,P_0,Q,R,PHI,DELTA,GAMMA,y,u,x_barprev,i_prev,P_prev)
[a,b]=size(P_0);
I=eye(a);
if i_prev ==0
    x_barnext=x_barprev;
    x_hat=x_barprev;
    P_next=P_0;
else
    %[kest,L,P,M,Z]=kalmd(sys,Q_kalman,R_kalman,h)
    K=P_prev*(H')*inv(H*P_prev*(H')+R);
    x_hat=x_barprev+K*(y-H*x_barprev);
    P_hat=(I-K*H)*P_prev*(I-K*H)'+K*R*K';
    
    x_barnext=PHI*x_hat+DELTA*u;
    P_next=PHI*P_hat*PHI'+GAMMA*Q*GAMMA';
end

i_next=i_prev+1;
end

== matlab function ModelSupervisor/Linerar System/theta system /MATLAB Function ==
  data: u input; w input; f input; x input; x_dot input; data input; theta input; theta_dotdot output
function theta_dotdot  = fcn(u, w, f, x, x_dot, data, theta)
L = data(1);
M = data(2);
m = data(3);
b = data(4);
k = data(5);
g = data(6);

% theta = theta * 180 / pi;

theta_dotdot=(-u + w + (m + M) * g * theta - (M / m) * f + b * x_dot + k * x)/(L * M);

end

== matlab function ModelSupervisor/Nonlinear system /calculating x_dot_dot ==
  data: C input; u input; x_dotdot output; w input; f input; x input; x_dot input; theta input; theta_dot input; theta_dotdot output
function [x_dotdot, theta_dotdot]= fcn(C,u, w, f, x, x_dot, theta, theta_dot)
%extracting the know parameters from vector C
L = C(1); 
M= C(2); 
m=C(3); 
b = C(4); 
k = C(5); 
g = C(6);

%calculating x_dot_dot
 x_dotdot = (u - f - w + f*cos(theta)^2 ...
            + m*L*theta_dot^2*sin(theta) ...
            -m*g*sin(theta)*cos(theta)...
            -b*x_dot -k*x )/(M + m*sin(theta)^2); 

%calculating theta_dot_dot
 theta_dotdot = (-u*cos(theta)+w*cos(theta)...
                   -M*L*theta_dot^2*sin(theta)*cos(theta)...
                    +(m+M)*g*sin(theta)-(M/m)*f*cos(theta)...
                    +b*x_dot*cos(theta)...
                    + k*x*cos(theta))/(L*(M+m*sin(theta)^2));

== matlab function ModelSupervisor/KalmanFilter1/KalmanBlock1/Klaman ==
  data: H input; P_0 input; Q input; R input; PHI input; DELTA input; GAMMA input; y input; u input; x_barprev input; i_prev input; P_prev input; x_hat output; x_barnext output; i_next output; P_next output
function [x_hat,x_barnext,i_next,P_next] = KalmanFilter(H,P_0,Q,R,PHI,DELTA,GAMMA,y,u,x_barprev,i_prev,P_prev)
[a,b]=size(P_0);
I=eye(a);
if i_prev ==0
    x_barnext=x_barprev;
    x_hat=x_barprev;
    P_next=P_0;
else
    %[kest,L,P,M,Z]=kalmd(sys,Q_kalman,R_kalman,h)
    K=P_prev*(H')*inv(H*P_prev*(H')+R);
    x_hat=x_barprev+K*(y-H*x_barprev);
    P_hat=(I-K*H)*P_prev*(I-K*H)'+K*R*K';
    
    x_barnext=PHI*x_hat+DELTA*u;
    P_next=PHI*P_hat*PHI'+GAMMA*Q*GAMMA';
end

i_next=i_prev+1;
end

== matlab function ModelSupervisor/KalmanFilter/KalmanBlock3/Klaman ==
  data: H input; P_0 input; Q input; R input; PHI input; DELTA input; GAMMA input; y input; u input; x_barprev input; i_prev input; P_prev input; x_hat output; x_barnext output; i_next output; P_next output
function [x_hat,x_barnext,i_next,P_next] = KalmanFilter(H,P_0,Q,R,PHI,DELTA,GAMMA,y,u,x_barprev,i_prev,P_prev)
[a,b]=size(P_0);
I=eye(a);
if i_prev ==0
    x_barnext=x_barprev;
    x_hat=x_barprev;
    P_next=P_0;
else
    %[kest,L,P,M,Z]=kalmd(sys,Q_kalman,R_kalman,h)
    K=P_prev*(H')*inv(H*P_prev*(H')+R);
    x_hat=x_barprev+K*(y-H*x_barprev);
    P_hat=(I-K*H)*P_prev*(I-K*H)'+K*R*K';
    
    x_barnext=PHI*x_hat+DELTA*u;
    P_next=PHI*P_hat*PHI'+GAMMA*Q*GAMMA';
end

i_next=i_prev+1;
end

== matlab function ModelSupervisor/KalmanFilter/KalmanBlock2/Klaman ==
  data: H input; P_0 input; Q input; R input; PHI input; DELTA input; GAMMA input; y input; u input; x_barprev input; i_prev input; P_prev input; x_hat output; x_barnext output; i_next output; P_next output
function [x_hat,x_barnext,i_next,P_next] = KalmanFilter(H,P_0,Q,R,PHI,DELTA,GAMMA,y,u,x_barprev,i_prev,P_prev)
[a,b]=size(P_0);
I=eye(a);
if i_prev ==0
    x_barnext=x_barprev;
    x_hat=x_barprev;
    P_next=P_0;
else
    %[kest,L,P,M,Z]=kalmd(sys,Q_kalman,R_kalman,h)
    K=P_prev*(H')*inv(H*P_prev*(H')+R);
    x_hat=x_barprev+K*(y-H*x_barprev);
    P_hat=(I-K*H)*P_prev*(I-K*H)'+K*R*K';
    
    x_barnext=PHI*x_hat+DELTA*u;
    P_next=PHI*P_hat*PHI'+GAMMA*Q*GAMMA';
end

i_next=i_prev+1;
end

== matlab function ModelSupervisor/KalmanFilter/KalmanBlock1/Klaman ==
  data: H input; P_0 input; Q input; R input; PHI input; DELTA input; GAMMA input; y input; u input; x_barprev input; i_prev input; P_prev input; x_hat output; x_barnext output; i_next output; P_next output
function [x_hat,x_barnext,i_next,P_next] = KalmanFilter(H,P_0,Q,R,PHI,DELTA,GAMMA,y,u,x_barprev,i_prev,P_prev)
[a,b]=size(P_0);
I=eye(a);
if i_prev ==0
    x_barnext=x_barprev;
    x_hat=x_barprev;
    P_next=P_0;
else
    %[kest,L,P,M,Z]=kalmd(sys,Q_kalman,R_kalman,h)
    K=P_prev*(H')*inv(H*P_prev*(H')+R);
    x_hat=x_barprev+K*(y-H*x_barprev);
    P_hat=(I-K*H)*P_prev*(I-K*H)'+K*R*K';
    
    x_barnext=PHI*x_hat+DELTA*u;
    P_next=PHI*P_hat*PHI'+GAMMA*Q*GAMMA';
end

i_next=i_prev+1;
end

== matlab function ModelSupervisor/KalmanFilter/DHT/MATLAB Function ==
  data: x_hat input; y input; Prob output; C input; R input; P input; Prob_prev input
function Prob  = fcn(x_hat, y, C, R, P, Prob_prev)

Prob_tot = 0;
Prob_0 = zeros(4, 1);
lower_bound = 10e-10;

for i = 1:4
    x_hat_i = x_hat(1 + 6*(i-1) : 6 + 6*(i-1));
    P_i = P(:, 1 + 6*(i-1) : 6 + 6*(i-1));
    
    y_tilde = y - C * x_hat_i;
    S = C * P_i * C' + R;
    Prob_0(i) = Prob_prev(i) * exp(-0.5*y_tilde' * inv(S) * y_tilde)/ ...
        (sqrt((2*pi)^3 * norm(S)));
    
    Prob_tot = Prob_tot + Prob_0(i);
end

Prob = max(lower_bound, Prob_0 ./ Prob_tot);
end

== matlab function ModelSupervisor/KalmanFilter1/KalmanBlock2/Klaman ==
  data: H input; P_0 input; Q input; R input; PHI input; DELTA input; GAMMA input; y input; u input; x_barprev input; i_prev input; P_prev input; x_hat output; x_barnext output; i_next output; P_next output
function [x_hat,x_barnext,i_next,P_next] = KalmanFilter(H,P_0,Q,R,PHI,DELTA,GAMMA,y,u,x_barprev,i_prev,P_prev)
[a,b]=size(P_0);
I=eye(a);
if i_prev ==0
    x_barnext=x_barprev;
    x_hat=x_barprev;
    P_next=P_0;
else
    %[kest,L,P,M,Z]=kalmd(sys,Q_kalman,R_kalman,h)
    K=P_prev*(H')*inv(H*P_prev*(H')+R);
    x_hat=x_barprev+K*(y-H*x_barprev);
    P_hat=(I-K*H)*P_prev*(I-K*H)'+K*R*K';
    
    x_barnext=PHI*x_hat+DELTA*u;
    P_next=PHI*P_hat*PHI'+GAMMA*Q*GAMMA';
end

i_next=i_prev+1;
end

== matlab function ModelSupervisor/KalmanFilter1/KalmanBlock3/Klaman ==
  data: H input; P_0 input; Q input; R input; PHI input; DELTA input; GAMMA input; y input; u input; x_barprev input; i_prev input; P_prev input; x_hat output; x_barnext output; i_next output; P_next output
function [x_hat,x_barnext,i_next,P_next] = KalmanFilter(H,P_0,Q,R,PHI,DELTA,GAMMA,y,u,x_barprev,i_prev,P_prev)
[a,b]=size(P_0);
I=eye(a);
if i_prev ==0
    x_barnext=x_barprev;
    x_hat=x_barprev;
    P_next=P_0;
else
    %[kest,L,P,M,Z]=kalmd(sys,Q_kalman,R_kalman,h)
    K=P_prev*(H')*inv(H*P_prev*(H')+R);
    x_hat=x_barprev+K*(y-H*x_barprev);
    P_hat=(I-K*H)*P_prev*(I-K*H)'+K*R*K';
    
    x_barnext=PHI*x_hat+DELTA*u;
    P_next=PHI*P_hat*PHI'+GAMMA*Q*GAMMA';
end

i_next=i_prev+1;
end

== matlab function ModelSupervisor/KalmanFilter1/KalmanBlock4/Klaman ==
  data: H input; P_0 input; Q input; R input; PHI input; DELTA input; GAMMA input; y input; u input; x_barprev input; i_prev input; P_prev input; x_hat output; x_barnext output; i_next output; P_next output
function [x_hat,x_barnext,i_next,P_next] = KalmanFilter(H,P_0,Q,R,PHI,DELTA,GAMMA,y,u,x_barprev,i_prev,P_prev)
[a,b]=size(P_0);
I=eye(a);
if i_prev ==0
    x_barnext=x_barprev;
    x_hat=x_barprev;
    P_next=P_0;
else
    %[kest,L,P,M,Z]=kalmd(sys,Q_kalman,R_kalman,h)
    K=P_prev*(H')*inv(H*P_prev*(H')+R);
    x_hat=x_barprev+K*(y-H*x_barprev);
    P_hat=(I-K*H)*P_prev*(I-K*H)'+K*R*K';
    
    x_barnext=PHI*x_hat+DELTA*u;
    P_next=PHI*P_hat*PHI'+GAMMA*Q*GAMMA';
end

i_next=i_prev+1;
end

== matlab function ModelSupervisor/KalmanFilter1/Subsystem3/MATLAB Function ==
  data: x_hat input; Prob output; C input; R input; P input; Prob_prev input
function Prob  = fcn(x_hat,C,R,P,Prob_prev)
for i =1:4
if  Prob_prev(i)<=10e-5 || isnan(Prob_prev(i))==1
             Prob_prev(i)=10e-5;
end
end       

Prob_1=0;
y_tilde=zeros(2,4);
S=zeros(2,8);
Prob_0=zeros(4,1);

for i =1:4
    y_tilde(:,i)=C * x_hat(1+6*(i-1):6+6*(i-1));
    S(:,1+2*(i-1):2+2*(i-1))=C*P(:,1+6*(i-1):6+6*(i-1))*C'+R;
    Prob_0(i)=exp(-0.5*y_tilde(:,i)'*inv(S(i))*y_tilde(:,i))/(sqrt((2*pi)^3*abs(S(i))));
    
        if  Prob_0(i)<=10e-5 || isnan(Prob_0(i))==1
             Prob_0(i)=10e-5;
        end
   
    
    Prob_1=Prob_1+Prob_0(i)*Prob_prev(i);

end

Prob= (Prob_0./Prob_1) .* Prob_prev;



end

== matlab function ModelSupervisor/KalmanFilter/DHT1/MATLAB Function ==
  data: x_hat input; y input; Prob output; C input; R input; P1 input; P2 input; P3 input; P4 input; Prob_prev input; Prob_0 output; y output
function [Prob, Prob_0, y]  = fcn(x_hat, y, C, R, P1, P2, P3, P4, Prob_prev)

% Prob_tot = 0;
% Prob_0 = zeros(4, 1);
% lower_bound = 10e-6;
% 
% for i = 1:4
%     x_hat_i = x_hat(1 + 6*(i-1) : 6 + 6*(i-1));
%     P_i = eye(6); % Hack to make Simulink accept the switch statement
%     switch(i)
%         case 1
%             P_i = P1;
%         case 2
%             P_i = P2;
%         case 3
%             P_i = P3;
%         case 4
%             P_i = P4;
%     end
%     
%     y_tilde = y - C * x_hat_i;
%     S = C * P_i * C' + R;
%     Prob_0(i) = exp(-0.5*y_tilde' * inv(S) * y_tilde)/(sqrt((2*pi)^3 * det(S)));
%     
%     if  Prob_0(i) <= lower_bound || isnan(Prob_0(i))
%         Prob_0(i) = lower_bound;
%     end
%     
%     
%     Prob_tot = Prob_tot + Prob_0(i) * Prob_prev(i);
%     
% end
% 
% Prob = (Prob_0 ./ Prob_tot) .* Prob_prev;

% function p_out  = DHT(y_tilde1,y_tilde2,y_tilde3,y_tilde4,S1,S2,S3,S4,p_in)

y_tilde = cell(1, 4);


for i = 1:4
    x_hat_i = x_hat(1 + 6*(i-1) : 6 + 6*(i-1));
    y_tilde{i} = y - C * x_hat_i;
end

S1 = C * P1 * C' + R;
S2 = C * P2 * C' + R;
S3 = C * P3 * C' + R;
S4 = C * P4 * C' + R;

minVariable = 10^-10;

temp = zeros(4,1);
Prob = zeros(4,1);

temp(1) = Prob_prev(1)*exp(-0.5*y_tilde{1}'*inv(S1)*y_tilde{1})/sqrt((2*pi)^3*norm(S1));
temp(2) = Prob_prev(2)*exp(-0.5*y_tilde{2}'*inv(S2)*y_tilde{2})/sqrt((2*pi)^3*norm(S2));
temp(3) = Prob_prev(3)*exp(-0.5*y_tilde{3}'*inv(S3)*y_tilde{3})/sqrt((2*pi)^3*norm(S3));
temp(4) = Prob_prev(4)*exp(-0.5*y_tilde{4}'*inv(S4)*y_tilde{4})/sqrt((2*pi)^3*norm(S4));

sum = temp(1) + temp(2) + temp(3) + temp(4);

Prob(1) = max(minVariable,temp(1)/sum);
Prob(2) = max(minVariable,temp(2)/sum);
Prob(3) = max(minVariable,temp(3)/sum);
Prob(4) = max(minVariable,temp(4)/sum);

Prob_0 = [temp(1), temp(2), temp(3), temp(4)];

end

== matlab function ModelSupervisor/Nonlinear system /Supervisor/Supervisor ==
  data: probs input; ctrl_selection output; current_time input; current_controller input; last_change_time input; last_change_time output
function [ctrl_selection, last_change_time] = supervisor( ...
probs, current_time, current_controller, last_change_time )

min_interval = 0.005; % Dwell time

[~, best_controller] = max(probs);

if current_time - last_change_time > min_interval
    current_controller = best_controller;
    last_change_time = current_time;
end

ctrl_selection = current_controller;

end
